simulink model "VSC_GFo_Fixed_Frequency_wi_LCL_v2017b"  (R2017b)
settings: Solver=ode1  StartTime=0.0  StopTime=10  FixedStep=Time_Step  MaxStep=1e-5  RelTol=1e-3
values from neighbouring files (symbols this model uses):
  fb = fn    (= 50)    [VSC_GFo_Init.m]    (also in VSC_GFo_Init_v1.m; VSC_GFo_Init_wi_LCL.m)
  fn = 50    [VSC_GFo_Init.m]    (also in VSC_GFo_Init_v1.m; VSC_GFo_Init_wi_LCL.m)
  GRD00_H = 5    [VSC_GFo_Init.m]    (also in VSC_GFo_Init_v1.m; VSC_GFo_Init_wi_LCL.m)
  GRD00_R = 4/100    (= 0.04)    [VSC_GFo_Init.m]    (also in VSC_GFo_Init_v1.m; VSC_GFo_Init_wi_LCL.m)
  GRD00_TD = 6    [VSC_GFo_Init.m]    (also in VSC_GFo_Init_v1.m = 2; VSC_GFo_Init_wi_LCL.m = 2)
  GRD00_TN = 1    [VSC_GFo_Init.m]    (also in VSC_GFo_Init_v1.m; VSC_GFo_Init_wi_LCL.m)
  GRD00_Ub = GRD00_Un    (= 400000)    [VSC_GFo_Init.m]    (also in VSC_GFo_Init_v1.m; VSC_GFo_Init_wi_LCL.m)
  Time_Step = 40e-6    (= 4e-05)    [VSC_GFo_Init.m]    (also in VSC_GFo_Init_v1.m; VSC_GFo_Init_wi_LCL.m)
  VSC01_Cf_pu = 0.066    [VSC_GFo_Init.m]    (also in VSC_GFo_Init_wi_LCL.m)
  VSC01_Lf_pu = 0.15    [VSC_GFo_Init.m]    (also in VSC_GFo_Init_wi_LCL.m)
  VSC01_Lt_pu = 0.15    [VSC_GFo_Init.m]    (also in VSC_GFo_Init_v1.m; VSC_GFo_Init_wi_LCL.m)
  VSC01_mp1 = 0.0043    [VSC_GFo_Init.m]    (also in VSC_GFo_Init_v1.m; VSC_GFo_Init_wi_LCL.m)
  VSC01_mp2 = 0.003    [VSC_GFo_Init.m]    (also in VSC_GFo_Init_v1.m = 0.0033; VSC_GFo_Init_wi_LCL.m = 0.0033)
  VSC01_mp3 = 0.04    [VSC_GFo_Init.m]    (also in VSC_GFo_Init_v1.m; VSC_GFo_Init_wi_LCL.m)
  VSC01_Pn = 1000 * 1e6    (= 1000000000)    [VSC_GFo_Init.m]    (also in VSC_GFo_Init_v1.m; VSC_GFo_Init_wi_LCL.m)
  VSC01_R = 4/100    (= 0.04)    [VSC_GFo_Init.m]    (also in VSC_GFo_Init_v1.m; VSC_GFo_Init_wi_LCL.m)
  VSC01_Rt_pu = 0.005    [VSC_GFo_Init.m]    (also in VSC_GFo_Init_v1.m; VSC_GFo_Init_wi_LCL.m)
  VSC01_Rv = 0.09    [VSC_GFo_Init.m]    (also in VSC_GFo_Init_v1.m; VSC_GFo_Init_wi_LCL.m)
  VSC01_Sn = VSC01_Pn/VSC01_cosPhi_n    [VSC_GFo_Init.m]    (also in VSC_GFo_Init_v1.m; VSC_GFo_Init_wi_LCL.m)
  VSC01_T1 = 0.121    [VSC_GFo_Init.m]    (also in VSC_GFo_Init_v1.m; VSC_GFo_Init_wi_LCL.m)
  VSC01_T2 = 0.022    [VSC_GFo_Init.m]    (also in VSC_GFo_Init_v1.m; VSC_GFo_Init_wi_LCL.m)
  VSC01_Tr_PLL = 0.010    (= 0.01)    [VSC_GFo_Init.m]    (also in VSC_GFo_Init_v1.m; VSC_GFo_Init_wi_LCL.m)
  VSC01_Udc_n = 640 * 1e3    (= 640000)    [VSC_GFo_Init.m]    (also in VSC_GFo_Init_v1.m; VSC_GFo_Init_wi_LCL.m)
  VSC01_Udcb = VSC01_Udc_n    (= 640000)    [VSC_GFo_Init.m]    (also in VSC_GFo_Init_v1.m; VSC_GFo_Init_wi_LCL.m)
  VSC01_Un1 = 320 * 1e3    (= 320000)    [VSC_GFo_Init.m]    (also in VSC_GFo_Init_v1.m; VSC_GFo_Init_wi_LCL.m)
  VSC01_Un2 = 400 * 1e3    (= 400000)    [VSC_GFo_Init.m]    (also in VSC_GFo_Init_v1.m; VSC_GFo_Init_wi_LCL.m)
  VSC01_W_LF = 60    [VSC_GFo_Init.m]    (also in VSC_GFo_Init_v1.m; VSC_GFo_Init_wi_LCL.m)
  VSC01_wc1 = wb/10    (= 31.4159265359)    [VSC_GFo_Init.m]    (also in VSC_GFo_Init_v1.m; VSC_GFo_Init_wi_LCL.m)
  VSC01_wc2 = 33.3    [VSC_GFo_Init.m]    (also in VSC_GFo_Init_v1.m; VSC_GFo_Init_wi_LCL.m)
  VSC01_wc3 = 2.5    [VSC_GFo_Init.m]    (also in VSC_GFo_Init_v1.m; VSC_GFo_Init_wi_LCL.m)
undefined symbols (not defined in the file or in its folder): C_line, VSC01_id0
libraries: powerlib x31, powerlib_meascontrol x1
(part 1 of 3)
settings Model: Creator=Frederic_Colas  LastModifiedBy=Frederic_Colas
settings OptimizationCC: LifeSpan=inf
settings DebuggingCC: UnconnectedInputMsg=none  UnconnectedOutputMsg=none  UnconnectedLineMsg=none  SFExecutionAtInitializationDiag=none
settings HardwareCC: ProdBitPerSizeT=32  ProdBitPerPtrDiffT=32  ProdWordSize=32  ProdHWDeviceType=Specified
settings CodeAppCC: StateflowObjectComments=on
settings SimscapeCC: SimscapeNormalizeSystem=off

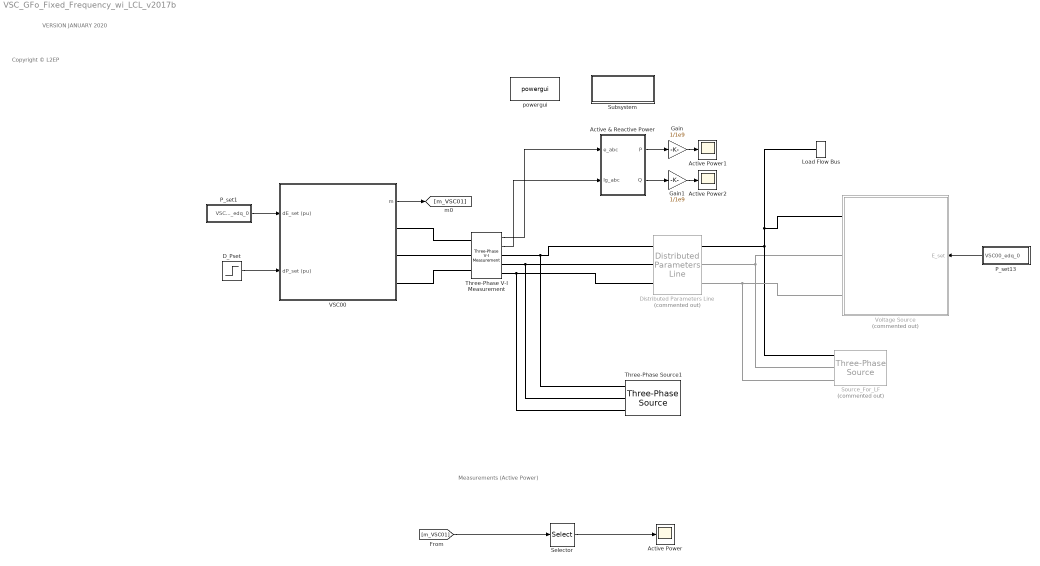
== system VSC_GFo_Fixed_Frequency_wi_LCL_v2017b ==
  note: VERSION JANUARY 2020
  note: Measurements (Active Power)
  note: Copyright © L2EP
  " Active & Reactive Power" : Subsystem  DialogController=POWERSYS.PowerSysDialog
  Active Power : Scope
  Active Power1 : Scope
  Active Power2 : Scope
  D_Pset : Step  Time=3  After=0.5  SampleTime=0
  Distributed Parameters Line : powerlib/Elements/Distributed Parameters Line  Commented=on  Phases=3  Frequency=50  Resistance=[0.01273 0.3864]  Inductance="[0.9337e-3  4.1264e-3]"  Capacitance=[12.74e-9 7.751e-9]  Length=50  x1=[-0.00032 2.39913762382152e-07 0 0;-0.00028 2.40449608965266e-07 0 0;-0.00024 2.40947485767745e-07 0 0;-0.0002 2.41407314169069e-07 189243.062485438 -353216.120618855;-0.00016 2.41829021557003e-07 193666.648507906 -350810.196287985;-0.00012 2.42212541339063e-07 198059.65232152 -348348.874960401;-8e-05 2.42557812953028e-07 202421.380220051 -345832.545307272;-4e-05 2.42864781876509e-07 206751.143436103 -343261.604686222]  x2=[-0.00032 -5.84182066675362e-12 0 0;-0.00028 -5.11361265966804e-12 0 0;-0.00024 -4.38459715386461e-12 0 0;-0.0002 -3.65488926934273e-12 177854.071673971 -358284.704095765;-0.00016 -2.92460423543639e-12 182342.2489454 -356021.494083621;-0.00012 -2.1938573726182e-12 186801.632261942 -353702.064150429;-8e-05 -1.46276407428886e-12 191231.517435277 -351326.780561063;-4e-05 -7.31439788555296e-13 195631.204935183 -348896.018400338]  x3=[-0.00032 -6.2867245833204e-11 0 0;-0.00028 -1.06466715946698e-10 0 0;-0.00024 -1.50049373731543e-10 0 0;-0.0002 -1.93608336980848e-10 284.201133471447 -561.76295681645;-0.00016 -2.37136727229364e-10 291.237829865103 -558.147319596773;-0.00012 -2.80627670839675e-10 298.228536429288 -554.443544445083;-8e-05 -3.24074300087621e-10 305.172149250395 -550.652216230411;-4e-05 -3.67469754246795e-10 312.067571851468 -546.773933647434]  x4=[-0.00032 3.8186796224243e-10 0 0;-0.00028 4.26357649227894e-10 0 0;-0.00024 4.70780009398051e-10 0 0;-0.0002 5.15128027947269e-10 998.290466477195 -2098.49155462395;-0.00016 5.59394701809321e-10 1024.58137422879 -2085.7813087356;-0.00012 6.03573040763248e-10 1050.71048870407 -2072.74169379946;-8e-05 6.47656068537197e-10 1076.67368381297 -2059.37476892188;-4e-05 6.91636823910058e-10 1102.46685966599 -2045.68264489526]  x5=0.000282770783497871  V1=ones(3,3)  V2=ones(3,3)  I1=ones(3,3)  I2=ones(3,3)  nHarmo=1  Measurements=None
      settings: SourceProductName=Simscape Power Systems
  Gain : Gain  Gain=1/1e9
  Gain1 : Gain  Gain=1/1e9
  Load Flow Bus : powerlib/Measurements/Load Flow Bus  LConnTagsString=a  Phases=single  Connectors=on one side  ID=BUS_1  Vbase=400000  Vref=1  Vangle=0  VLF=1  VLFb=1  VLFc=1  angleLF=0  angleLFb=0  angleLFc=0
      settings: SourceProductName=Simscape Electrical
  P_set1 : Subsystem
  P_set13 : Subsystem
  Selector : Selector  InputPortWidth=3  IndexOptions=Index vector (dialog)  Indices=[1]  OutputSizes=1
  Source_For_LF : powerlib/Electrical Sources/Three-Phase Source  Commented=on  InternalConnection=Yg  VoltagePhases=off  Voltage=(400000)*1  PhaseAngle=0  Voltage_phases=[25e3 25e3 25e3]/sqrt(3)  PhaseAngles_phases=[0 -120 +120]  Frequency=fb  NonIdealSource=on  SpecifyImpedance=off  Resistance=0  Inductance=0  ShortCircuitLevel=100e6  BaseVoltage=GRD00_Un  XRratio=7  BusType=swing  Pref=P0  Qref=Q0  Prefabc=[10e3, 10e3, 10e3]  Qrefabc=[0, 0, 0]  Qmin=-inf  Qmax=inf
      settings: SourceProductName=Simscape Electrical
  Subsystem : Subsystem
      settings: OpenFcn=LoadFlow_VSC
      mask Display: color('blue'),disp('Update Loadflow')
  Three-Phase V-I Measurement : powerlib/Measurements/Three-Phase V-I Measurement  VoltageMeasurement=phase-to-ground  SetLabelV=off  LabelV=Vabc  Vpu=off  VpuLL=off  CurrentMeasurement=yes  SetLabelI=off  LabelI=Iabc  Ipu=off  Pbase=100e6  Vbase=500e3  OutputType=Complex  PhasorSimulation=off  PSBequivalent=0
  Three-Phase Source1 : powerlib/Electrical Sources/Three-Phase Source  InternalConnection=Yg  VoltagePhases=off  Voltage=(400000)*1  PhaseAngle=0  Voltage_phases=[25e3 25e3 25e3]/sqrt(3)  PhaseAngles_phases=[0 -120 +120]  Frequency=50  NonIdealSource=off  SpecifyImpedance=off  Resistance=0.8929  Inductance=16.58e-3  ShortCircuitLevel=100e6  BaseVoltage=25e3  XRratio=7  BusType=swing  Pref=10e3  Qref=0  Prefabc=[10e3, 10e3, 10e3]  Qrefabc=[0, 0, 0]  Qmin=-inf  Qmax=inf
  VSC00 : Subsystem  mask(VSC){fb=fb, Sn=VSC01_Sn, Pn=VSC01_Pn, Un1=VSC01_Un1, Un2=VSC01_Un2, Rt_pu=VSC01_Rt_pu, Lt_pu=VSC01_Lt_pu, Lm_pu=500, Rm_pu=500, Lf_pu=0.15, Cf_pu=0.066, Tr_PLL=VSC01_Tr_PLL, Tr_i=0, D_i=0, Tr_v=0, D_v=0, Val_Freq_Support=on, R_percent=VSC01_R, Rv=VSC01_Rv, W_TVR=VSC01_W_LF, gainpopup=2, wc1=VSC01_wc1, mp1=VSC01_mp1, wc2=VSC01_wc2, mp2=VSC01_mp2, wc3=VSC01_wc3, mp3=VSC01_mp3, T1=VSC01_T1, T2=VSC01_T2, LFpopup=PQ, P0=0.3, Q0=0, V0=1, Theta0=0}
      mask prompts: fb "Nominal Frequency (Hz)"; Sn "Nominal Apparent Power (VA)"; Pn "Nominal Power (W)"; Un1 "VSC side Nominal Ph-Ph Voltage (V)"; Un2 "Grid side Nominal Ph-Ph Voltage (V)"; Rt_pu "R (pu)"; Lt_pu "L (pu)"; Lm_pu "Rm (pu)"; Rm_pu "Lm (pu)"; Lf_pu "Lf (pu)"; Cf_pu "Cf (pu)"; Tr_PLL "PLL Time response (s)"; Tr_i "Time Response (s)"; D_i "Damping factor"; Tr_v "Time Response (s)"; D_v "Damping factor"; Val_Freq_Support "Frequency Support"; R_percent "Droop Gain (%)"; Rv "Damping Resistance (Rv)"; W_TVR "Dr filter"; gainpopup "Strategy"; wc1 "wc"; mp1 "mp"; wc2 "wc"; mp2 "mp"; wc3 "wc"; mp3 "mp"; P0 "Initial Active Power (pu)"; Q0 "Initial Reactive Power (pu)"; V0 "Initial Voltage (pu)"; Theta0 "Initial Angle (°)"
      mask init:
      | % Update Name of LF bus for internal purpose
      |     NameStr = [get_param(gcb,'Name')];% '_LF'];
      |     set_param([gcb '/Load Flow Bus'],'ID',NameStr);
      |     %disp(NameStr);
      |     
      | % Increase size of Mask dialog box
      |    % pause(0.1);
      |     
      |     
      | % Base values
      |     %Un = Un1;
      |     Pb = Pn;
      |     cos_phi_n = Pn/Sn;
      |     Sb = Pb/cos_phi_n;
      |     %Ub = Un;
      |     Vn = Un1/sqrt(3);
      |     Vb = Vn;
      |     Vn2 = Un2/sqrt(3);
      |     Vb2=Vn2;
      |     %Ib = Sb / Ub;
      |     Ib = Sb / (3*Vb);
      |     wb = 2*pi*fb;
      |     Zb = (Vb*sqrt(3))^2 / Sb;
      |     Lb = Zb / wb; % Inductance base value
      |     Cb = 1 / (Zb*wb); 
      |   
      | % PLL derivation of the parameters
      |     wn_PLL=5/Tr_PLL;
      |     zeta_PLL = 1;
      |     Kp_PLL_pu = 2*zeta_PLL*wn_PLL/wb;
      |     Ki_PLL_pu = wn_PLL^2/wb;
      | 
      |  %% Inner controller: Current & Voltage 
      | % Current PI controller   
      |     Tr_i = 5 * 1e-3;                    % Time response [s]
      |     D_i = 0.707;                        % Damping factor
      |     Kp_i = 0.73001;                     % Proportional current gain
      |     Ki_i = 1.19073;                     % Integral current gain
      |     Ti_i = Kp_i / Ki_i;
      |     
      |     Kffi = 1;                           % Current feed forward (enabled)  
      |  % Voltage PI controller   
      |     Tr_v = 5 * 1e-3;                    % Time response [s]
      |     D_v = 0.707;                        % Damping factor
      |     Kp_v = 0.52001;                     % Proportional current gain
      |     Ki_v = 1.16073;                     % Integral current gain
      |     Ti_iv = Kp_v / Ki_v;  
      |     Kffv = 1;                           % Current feed forward (enabled)     
      | % Set the chosen strategy
      |     Chosen_Strategy = str2double(gainpopup);
      |     
      | % Set the frequency droop gain
      |     R = R_percent;
      | 
      | % Compute Initial Voltage of VSC 
      | %   from steady-state output transformer model and Loadflow result
      |     if (LFpopup == 'PQ')
      |         V0 = 1;
      |     end
      | %%%%%%%%%%%%%%%%%%%        
      | %     R1_pu = Rt_pu/2;
      | %     L1_pu = Lt_pu/2;
      | %     R2_pu = Rt_pu/2;
      | %     L2_pu = Lt_pu/2;
      | %     X1_pu = L1_pu;
      | %     X2_pu = L2_pu;
      | %     Xm_pu = Lm_pu;
      | %     Zm_pu = 1/(1/Rm_pu+1/(1i*Xm_pu));
      | %     S0=P0+1i*Q0;
      | %     I2 = conj(S0)/(V0);
      | %     Vm = (R2_pu+1i*X2_pu)*I2 + V0;
      | %     Im = Vm/Zm_pu;
      | %     I1 = I2 + Im;
      | %     V1 = (R1_pu+1i*X1_pu) * I1 + Vm;
      | %     Vvsc0 = abs(V1);
      | %    % disp(Vvsc0*1000)
      | %     Theta_vsc0 = angle(V1) * 180/pi+Theta0;
      | %%%%%%%%%%%%%%%%%%%
      | %Rf_pu=0.005;
      | %Lf_pu=0.15;
      | %Cf_pu = 0.066;
      | %%%%%%%%%%%%%%%%%%%        
      |     R1_pu = (Rt_pu/2) ;
      |     L1_pu = (Lt_pu/2);
      |     R2_pu = Rt_pu/2;
      |     L2_pu = Lt_pu/2;
      |     X1_pu = L1_pu;
      |     X2_pu = L2_pu;
      |     Xm_pu = Lm_pu;
      |     Xc_pu = Cf_pu;
      |     Xf_pu = Lf_pu;
      |     Zt_pu = 1/(1/Rm_pu+1/(1i*Xm_pu));
      |     Zc_pu = 1/(1i*Xc_pu);
      |     S0=P0+1i*Q0; % Apparent output Power
      |     I2 = conj(S0)/(V0); % Output current
      |     %Vm = (R2_pu+1i*X2_pu)*I2 + V0;
      |     Vt = (R2_pu+1i*X2_pu) * I2 + V0; % Magnetizing Voltage
      |     %Vcf = (R2_pu+1i*X2_pu)*I2 + V0;
      |     It = Vt/Zt_pu; % Magnetizing current
      |     I1 = I2 + It; % output transformer Primary side current
      |     V1 = (R1_pu+1i*X1_pu) * I1 + Vt; % Output transformer Primary voltage = output capacitor voltage
      |     abs(V1)
      |     
      |     %LC Filter
      |     Im = I1 + 1i*Xc_pu*V1; % Converter output current
      |     Imd0 = abs(Im)*cos(angle(Im)-angle(V1));
      |     Imq0 = abs(Im)*sin(angle(Im)-angle(V1));
      |     Vm = 1i*Xf_pu*Im + V1; % Converter initial output voltage
      |     %Icf = Vcf/Zc_pu;
      |     %I1 = -It + Icf;
      |     %V1 = (Rf_pu+1i*Xf_pu) * I1 + Vcf;
      |     Vmd0 = abs(Vm)*cos(angle(Vm)-angle(V1));
      |     Vmq0 = abs(Vm)*sin(angle(Vm)-angle(V1));
      |     
      |     %Filtre LC
      |     
      |     Vvsc0 = abs(Vm)
      |     Theta_vsc0 = angle(Vm) * 180/pi+Theta0;
      | %%%%%%%%%%%%%%%%%%%
      | 
      | 
      |     %vd0=Vvsc0*cos(Theta0*2*pi/180);
      |     %vq0=Vvsc0*sin(Theta0*2*pi/180); 
      |  
      |     %Va0 = Vvsc0*sqrt(2)*Ub/sqrt(3)*sin(Theta_vsc0*pi/180);
      |     %Vb0 = Vvsc0*sqrt(2)*Ub/sqrt(3)*sin(Theta_vsc0*pi/180-2*pi/3);
      |     %Vc0 = Vvsc0*sqrt(2)*Ub/sqrt(3)*sin(Theta_vsc0*pi/180+2*pi/3);
      |     
      |     Va0 = Vvsc0*sqrt(2)*Vb*sin(Theta_vsc0*pi/180);
      |     Vb0 = Vvsc0*sqrt(2)*Vb*sin(Theta_vsc0*pi/180-2*pi/3);
      |     Vc0 = Vvsc0*sqrt(2)*Vb*sin(Theta_vsc0*pi/180+2*pi/3);
      |     
      | % Generate string to display LF results on Mask
      |     %str_tmp = fprintf("Vvsc0 = %d, Theta_vsc0 = %d°",Vvsc0,Theta_vsc0);
      |     mo = get_param(gcb,'MaskObject');
      |     mo.getDialogControl('LF_vsc_str').Prompt = ['V0 = ', num2str(Vvsc0),' pu, Angle = ', num2str(Theta_vsc0),'°'];
      |     mo.getDialogControl('LF_pcc_str').Prompt = ['V0 = ', num2str(V0),' pu, Angle = ', num2str(Theta0),'°'];
      |     mo.getDialogControl('LF_pcc_Power_str').Prompt = ['P0 = ', num2str(P0),' pu, Q0 = ', num2str(Q0),' pu'];
      |     %set_param([gcb],'LF_str',str_tmp);
      |  %GRD00_Theta0 = Theta0;
      |  %P0 = 200e6;
      |  %Q0 = 0;
      |  % Initial current values of VSC (dq pu) 
      |  %id0 =(P0*vd0+Q0*vq0)/(vd0^2+vq0^2) * 1/Ib; %
      |  %iq0 =(P0*vq0-Q0*vd0)/(vd0^2+vq0^2) * 1/Ib; %Initial current in the connexion inductance
      settings: OpenFcn=|
      | NameStr = get_param(gcb,'Name');
      | open_system(gcbh, 'Mask');
      | 
      | h2AllOpenDlgs = DAStudio.ToolRoot.getOpenDialogs;
      | 
      | for i=1:length(h2AllOpenDlgs)
      |     try
      |          %disp(h2AllOpenDlgs(i).getSource.getBlock.Name);
      |         Dialog_block_name = h2AllOpenDlgs(i).getSource.getBlock.Name;
      |          %strcmp(Dialog_block_name, NameStr),
      |         if (strcmp(h2AllOpenDlgs(i).getSource.getBlock.Name, NameStr))
      |             iPos = h2AllOpenDlgs(i).position;
      |             h2AllOpenDlgs(i).position = [iPos(1)   iPos(2)   iPos(3)*1.5   iPos(4)];
      |         end
      |     end
      | end
      mask TypeOptions gainpopup: 1 | 2 | 3
      mask Callback gainpopup:
      | % Get the mask parameter values. This is a cell
      | %   array of character vectors.
      | maskStr = get_param(gcb,'gainpopup');
      | p=Simulink.Mask.get(gcb);
      | 
      | % The pop-up menu is the first mask parameter.
      | %   Check the value selected in the pop-up
      | if strcmp(maskStr,'1'),
      | 
      |     % Set the visibility of both parameters on when
      |     %   User-defined is selected in the pop-up.
      |     p.getDialogControl('Param_Strat_1').Visible='on';
      |     p.getDialogControl('Param_Strat_2').Visible='off';
      |     p.getDialogControl('Param_Strat_3').Visible='off';
      | 
      | elseif strcmp(maskStr,'2'),
      | 
      |     % Set the visibility of both parameters on when
      |     %   User-defined is selected in the pop-up.
      |     p.getDialogControl('Param_Strat_1').Visible='off';
      |     p.getDialogControl('Param_Strat_2').Visible='on';
      |     p.getDialogControl('Param_Strat_3').Visible='off';
      | 
      |     % Turn off the visibility of the Value field
      |     %   when User-defined is not selected.
      | else
      | 
      |     % Set the visibility of both parameters on when
      |     %   User-defined is selected in the pop-up.
      |     p.getDialogControl('Param_Strat_1').Visible='off';
      |     p.getDialogControl('Param_Strat_2').Visible='off';
      |     p.getDialogControl('Param_Strat_3').Visible='on';
      | 
      | end
      mask TypeOptions LFpopup: Swing | PQ | PV
      mask Callback LFpopup:
      | % Get the mask parameter values. This is a cell
      | %   array of character vectors.
      | maskStr = get_param(gcb,'LFpopup');
      | p=Simulink.Mask.get(gcb);
      | 
      | % The pop-up menu is the first mask parameter.
      | %   Check the value selected in the pop-up
      | if strcmp(maskStr,'Swing'),
      | 
      |     % Set the visibility of both parameters on when
      |     %   User-defined is selected in the pop-up.
      |     p.getParameter('P0').Visible='off';
      |     p.getParameter('Q0').Visible='off';
      |     p.getParameter('V0').Visible='on';
      |     p.getParameter('Theta0').Visible='on';
      |     set_param([gcb '/Source_For_LF'],'BusType','swing');
      | 
      | elseif strcmp(maskStr,'PQ'),
      | 
      |     % Set the visibility of both parameters on when
      |     %   User-defined is selected in the pop-up.
      |     p.getParameter('P0').Visible='on';
      |     p.getParameter('Q0').Visible='on';
      |     p.getParameter('V0').Value='1';
      |     set_param(gcb,'V0','1');
      |     p.getParameter('V0').Visible='off';
      |     p.getParameter('Theta0').Visible='off';
      |     set_param([gcb '/Source_For_LF'],'BusType','PQ');
      | 
      |     % Turn off the visibility of the Value field
      |     %   when User-defined is not selected.
      | else
      | 
      |     % Set the visibility of both parameters on when
      |     %   User-defined is selected in the pop-up.
      |     p.getParameter('P0').Visible='on';
      |     p.getParameter('Q0').Visible='off';
      |     p.getParameter('V0').Visible='on';
      |     p.getParameter('Theta0').Visible='off';
      |     set_param([gcb '/Source_For_LF'],'BusType','PV');
      | 
      | end
      mask DialogControl Nominal_Param Prompt: Nominal Value
      mask DialogControl Container20 Prompt: Output Transformer
      mask DialogControl Container26 Prompt: Output Filter
      mask DialogControl Control_Param Prompt: Control Parameter
      mask DialogControl Container13 Prompt: Inner Control Parameters
      mask DialogControl Container27 Prompt: Current Loop
      mask DialogControl Container29 Prompt: Voltage Loop
      mask DialogControl Container14 Prompt: Frequency Support
      mask DialogControl Container15 Prompt: Transient Virtual Resistor
      mask DialogControl Container18 Prompt: Control Strategy
      mask DialogControl Title_Strat_1 Prompt: Strategy 1
      mask DialogControl Title_Strat_2 Prompt: Strategy 2
      mask DialogControl Title_Strat_3 Prompt: Strategy 3
      mask DialogControl LF_Param Prompt: Loadflow
      mask DialogControl Control4 Prompt: Initial Operating Point
      mask DialogControl Container24 Prompt: VSC side
      mask DialogControl LF_vsc_str Prompt: V0 = 0.9961 pu, Angle = 5.1844°
      mask DialogControl Container25 Prompt: PCC
      mask DialogControl LF_pcc_str Prompt: V0 = 1 pu, Angle = 0°
      mask DialogControl LF_pcc_Power_str Prompt: P0 = 0.3 pu, Q0 = 0 pu
      mask DialogControl UpdateLoadflow Prompt: Update Loadflow
      mask DialogControl UpdateLoadflow Callback: Load_Flow_VSC
  Voltage Source : Subsystem  Commented=on  mask(Inertial_Voltage_source){fb=fb, Sc=1e9, Ub=GRD00_Ub, H_eq=GRD00_H, Droop=GRD00_R, TN=GRD00_TN, TD=GRD00_TD}
      mask prompts: fb "Nominal Frequency (Hz)"; Sc "Nominal Power (VA)"; Ub "Nominal Voltage (V)"; H_eq "Inertial Constant H (s)"; Droop "Droop Gain"; TN "Lead Time Constant"; TD "Lag Time Constant"
      mask init:
      | % Base values
      |     wb=2*pi*fb;
      |     Ib=Sc/(sqrt(3)*Ub);
      |     Vb=Ub/sqrt(3);
      |     e0=Vb;
      |     Theta_e0=0;
      |   
      | % Parameters
      |     R=Droop;
      mask DialogControl Container5 Prompt: Nominal Values
      mask DialogControl Container16 Prompt: Network Time Constants
  powergui : powerlib/powergui  Priority=1  SimulationMode=Discrete  SampleTime=Time_Step  frequency=60  Iterations=100  frequencyindice=50  Pbase=1000e6  ErrMax=1e-5  UnitsV=kV  UnitsW=MW  buscounter=0  FunctionMessages=off  echomessages=off  EnableUseOfTLC=off  CurrentSourceSwitches=off  DisableSnubberDevices=off  DisableRonSwitches=off  DisableVfSwitches=off  DisplayEquations=off  SolverType=Tustin/Backward Euler (TBE)  Interpol=off  ExternalGateDelay=off  methode=off  Ts=100  x0status=blocks  SPID=on  SwTol=0  HookPort=off  RestoreLinks=warning  ResistiveCurrentMeasurement=off  Frange=[0:2:500]  Ylog=off  Xlog=on  ShowGrid=off  save=off  variable=ZData  structure=0  ZoomFFT=off  StartTime=0.0  cycles=1  DisplayStyle=1  fundamental=60  FreqAxis=off  MaxFrequency=1000  frequencyindicesteady=1  RmsSteady=1  display=off
  wires:
  P_set1/1(VSC01_edq_0) -> VSC00/1(dE_set (pu))
  D_Pset/1 -> VSC00/2(dP_set (pu))
  [m_VSC01] -> Selector/1
  P_set13/1(VSC00_edq_0) -> Voltage Source/1(E_set)
  Selector/1 -> Active Power/1
  VSC00/1(m) -> [m_VSC01]
  Three-Phase V-I Measurement/1 -> " Active & Reactive Power"/1(e_abc)
  Three-Phase V-I Measurement/2 -> " Active & Reactive Power"/2(Ig_abc)
  " Active & Reactive Power"/1(P) -> Gain/1
  " Active & Reactive Power"/2(Q) -> Gain1/1
  Gain/1 -> Active Power1/1
  Gain1/1 -> Active Power2/1
  connections:
  Source_For_LF/RConn2 -- Voltage Source/RConn2 -- Distributed Parameters Line/RConn2
  Voltage Source/RConn1 -- Source_For_LF/RConn1 -- Distributed Parameters Line/RConn1 -- Load Flow Bus/LConn1
  Source_For_LF/RConn3 -- Distributed Parameters Line/RConn3 -- Voltage Source/RConn3
  Three-Phase V-I Measurement/LConn2 -- VSC00/RConn2
  Three-Phase V-I Measurement/RConn2 -- Three-Phase Source1/RConn2 -- Distributed Parameters Line/LConn2
  Three-Phase V-I Measurement/RConn1 -- Distributed Parameters Line/LConn1 -- Three-Phase Source1/RConn1
  Three-Phase V-I Measurement/RConn3 -- Distributed Parameters Line/LConn3 -- Three-Phase Source1/RConn3
  Three-Phase V-I Measurement/LConn3 -- VSC00/RConn3
  Three-Phase V-I Measurement/LConn1 -- VSC00/RConn1

== system VSC_GFo_Fixed_Frequency_wi_LCL_v2017b/ Active & Reactive Power ==
  e_abc : Inport  PortDimensions=3
  Ig_abc : Inport  Port=2  PortDimensions=3
  Demux : Demux  Outputs=3
  Mux : Mux  Inputs=3
  Product1 : Product  SaturateOnIntegerOverflow=on  InputSameDT=on  OutDataTypeStr=Inherit: Same as first input
  Product3 : Product  SaturateOnIntegerOverflow=on  InputSameDT=on  OutDataTypeStr=Inherit: Same as first input
  Sum : Sum  Inputs=+-  SaturateOnIntegerOverflow=on  InputSameDT=on  OutDataTypeStr=Inherit: Same as first input
  Sum1 : Sum  Inputs=1  SaturateOnIntegerOverflow=on  InputSameDT=on  OutDataTypeStr=Inherit: Same as first input
  Sum4 : Sum  Inputs=1  SaturateOnIntegerOverflow=on  InputSameDT=on  OutDataTypeStr=Inherit: Same as first input
  Sum5 : Sum  Inputs=+-  SaturateOnIntegerOverflow=on  InputSameDT=on  OutDataTypeStr=Inherit: Same as first input
  Sum6 : Sum  Inputs=+-  SaturateOnIntegerOverflow=on  InputSameDT=on  OutDataTypeStr=Inherit: Same as first input
  pu->V : Gain  Gain=1/sqrt(3)  SaturateOnIntegerOverflow=on  OutDataTypeStr=Inherit: Same as input  ParamDataTypeStr=Inherit: Same as input
  P : Outport
  Q : Outport  Port=2
  wires:
  pu->V/1 -> Q/1  "Q"
  Mux/1 -> Product3/1
  Sum6/1 -> Mux/2
  Sum5/1 -> Mux/1
  Sum/1 -> Mux/3
  Demux/3 -> Sum6/1, Sum5/2
  Demux/2 -> Sum5/1, Sum/2
  Demux/1 -> Sum6/2, Sum/1
  Sum4/1 -> P/1  "P"
  Ig_abc/1 -> Product3/2, Product1/2
  e_abc/1 -> Demux/1, Product1/1
  Product1/1 -> Sum4/1
  Product3/1 -> Sum1/1
  Sum1/1 -> pu->V/1

== system VSC_GFo_Fixed_Frequency_wi_LCL_v2017b/P_set1 ==
  Mux : Mux  Inputs=2
  ed0 : Constant  Value=0
  eq0 : Constant  Value=0
  VSC01_edq_0 : Outport
  wires:
  eq0/1 -> Mux/2
  ed0/1 -> Mux/1
  Mux/1 -> VSC01_edq_0/1

== system VSC_GFo_Fixed_Frequency_wi_LCL_v2017b/P_set13 ==
  Mux : Mux  Inputs=2
  ed1 : Constant  Value=0
  eq1 : Constant
  VSC00_edq_0 : Outport
  wires:
  Mux/1 -> VSC00_edq_0/1
  eq1/1 -> Mux/1
  ed1/1 -> Mux/2

== system VSC_GFo_Fixed_Frequency_wi_LCL_v2017b/Subsystem ==

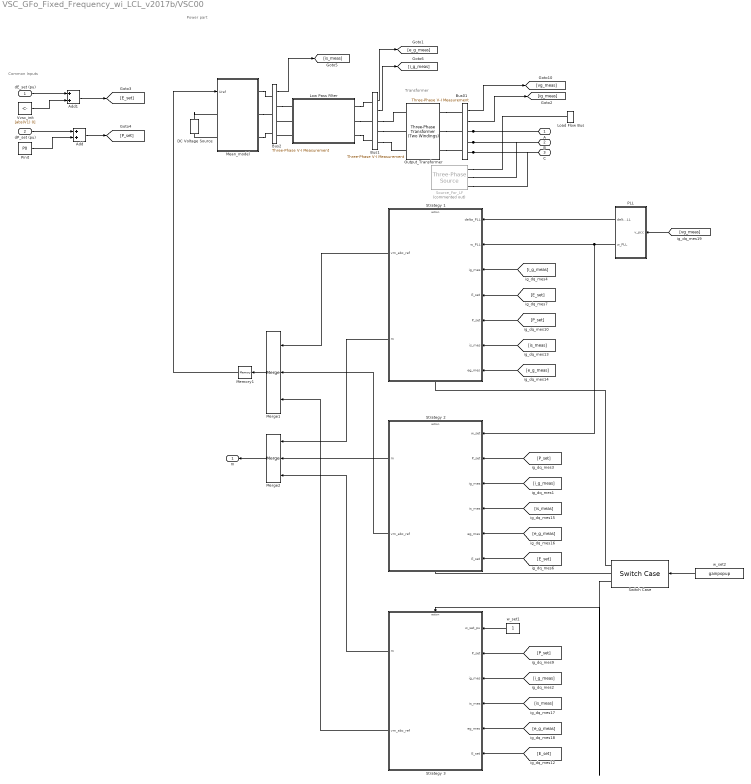
== system VSC_GFo_Fixed_Frequency_wi_LCL_v2017b/VSC00 ==
  note: Power part
  note: Common Inputs
  note: Transformer
  dE_set (pu) : Inport
  dP_set (pu) : Inport  Port=2
  Add : Sum
  Add1 : Sum
  Bus01 : powerlib/Measurements/Three-Phase V-I Measurement  VoltageMeasurement=phase-to-ground  SetLabelV=off  LabelV=Vabc  Vpu=off  VpuLL=off  CurrentMeasurement=yes  SetLabelI=off  LabelI=Iabc  Ipu=off  Pbase=100e6  Vbase=500e3  OutputType=Complex  PhasorSimulation=off  PSBequivalent=0
      settings: SourceProductName=Simscape Electrical
  Bus1 : powerlib/Measurements/Three-Phase V-I Measurement  VoltageMeasurement=phase-to-ground  SetLabelV=off  LabelV=Vabc  Vpu=off  VpuLL=off  CurrentMeasurement=yes  SetLabelI=off  LabelI=Iabc  Ipu=off  Pbase=100e6  Vbase=500e3  OutputType=Complex  PhasorSimulation=off  PSBequivalent=0
      settings: SourceProductName=Simscape Electrical
  Bus2 : powerlib/Measurements/Three-Phase V-I Measurement  VoltageMeasurement=no  SetLabelV=off  LabelV=Vabc  Vpu=off  VpuLL=off  CurrentMeasurement=yes  SetLabelI=off  LabelI=Iabc  Ipu=off  Pbase=100e6  Vbase=500e3  OutputType=Complex  PhasorSimulation=off  PSBequivalent=0
      settings: SourceProductName=Simscape Electrical
  DC Voltage Source : powerlib/Electrical Sources/DC Voltage Source  Amplitude=VSC01_Udc_n  Measurements=Voltage
      settings: SourceProductName=Simscape Electrical
  Load Flow Bus : powerlib/Measurements/Load Flow Bus  LConnTagsString=a  Phases=single  Connectors=on one side  ID=VSC00  Vbase=Un2  Vref=V0  Vangle=Theta0  VLF=1.002  VLFb=1  VLFc=1  angleLF=1.777  angleLFb=0  angleLFc=0
      settings: SourceProductName=Simscape Electrical
  Low Pass Filter : Subsystem
  Mean_model : Subsystem
  Memory1 : Memory  InitialCondition=[Va0 Vb0 Vc0]
  Merge1 : Merge  Inputs=3
  Merge2 : Merge  Inputs=3
  Output_Transformer : powerlib/Elements/Three-Phase Transformer (Two Windings)  Winding1Connection=Yg  Winding2Connection=Yg  CoreType=Three single-phase transformers  SetSaturation=off  Hysteresis=off  DataFile='hysteresis'  SetInitialFlux=off  Measurements=None  UNITS=pu  NominalPower=[Sn , fn ]  Winding1=[Un1 , Rt_pu/2 , Lt_pu/2]  Winding2=[Un2 , Rt_pu/2 , Lt_pu/2]  Rm=Rm_pu  Lm=Lm_pu  L0=0.5  Saturation=[ 0,0 ; 0.0024,1.2 ; 1.0,1.52 ]  InitialFluxes=[ 0.8 , -0.8 , 0.7 ]  MoreParameters=off  BreakLoop=off  DataType=off  TransfoNumber=1
      settings: SourceProductName=Simscape Electrical
  PLL : Subsystem
  Pinit : Constant  Value=P0
  Source_For_LF : powerlib/Electrical Sources/Three-Phase Source  Commented=on  InternalConnection=Yg  VoltagePhases=off  Voltage=(400000)*1.00234  PhaseAngle=1.7773  Voltage_phases=[25e3 25e3 25e3]/sqrt(3)  PhaseAngles_phases=[0 -120 +120]  Frequency=50  NonIdealSource=off  SpecifyImpedance=off  Resistance=0  Inductance=0  ShortCircuitLevel=100e6  BaseVoltage=Un  XRratio=7  BusType=PQ  Pref=P0*Sb  Qref=Q0*Sb  Prefabc=[10e3, 10e3, 10e3]  Qrefabc=[0, 0, 0]  Qmin=-inf  Qmax=inf
      settings: SourceProductName=Simscape Electrical
  Strategy 1 : Subsystem
  Strategy 2 : Subsystem
  Strategy 3 : Subsystem
  Switch Case : SwitchCase  CaseConditions={1,2,3}  ShowDefaultCase=off
  Vvsc_init : Constant  Value=[abs(V1) 0]
  w_set1 : Constant
  w_set2 : Constant  Value=gainpopup
  A : PMIOPort  Port=1  Side=Right
  B : PMIOPort  Port=2  Side=Right
  C : PMIOPort  Port=3  Side=Right
  m : Outport
  wires:
  PLL/1(delta_PLL) -> Strategy 1/1(delta_PLL)
  w_set1/1 -> Strategy 3/1(w_set_pu)
  Add/1 -> [P_set]
  Strategy 2/1(m) -> Merge2/2
  [i_g_meas] -> Strategy 1/3(ig_mes)
  Switch Case/1 -> Strategy 1/Action
  [vg_meas] -> PLL/1(v_pcc)
  Merge2/1 -> m/1
  Bus01/2 -> [ig_meas]
  dE_set (pu)/1 -> Add1/1
  Strategy 1/1(vm_abc_ref) -> Merge1/1
  Switch Case/3 -> Strategy 3/Action
  Strategy 1/2(m) -> Merge2/1
  w_set2/1 -> Switch Case/1
  Bus01/1 -> [vg_meas]
  [P_set] -> Strategy 3/2(P_set)
  Strategy 3/1(m) -> Merge2/3
  PLL/2(w_PLL) -> Strategy 2/1(w_set), Strategy 1/2(w_PLL)
  Add1/1 -> [E_set]
  [P_set] -> Strategy 2/2(P_set)
  Strategy 2/2(vm_abc_ref) -> Merge1/2
  Vvsc_init/1 -> Add1/2
  Merge1/1 -> Memory1/1
  [P_set] -> Strategy 1/5(P_set)
  Pinit/1 -> Add/2
  Switch Case/2 -> Strategy 2/Action
  dP_set (pu)/1 -> Add/1
  [E_set] -> Strategy 1/4(E_set)
  Memory1/1 -> Mean_model/1(Uref)
  Bus1/1 -> [e_g_meas]
  Bus2/1 -> [is_meas]
  [e_g_meas] -> Strategy 1/7(eg_mes)
  [is_meas] -> Strategy 1/6(is_mes)
  Bus1/2 -> [i_g_meas]
  [E_set] -> Strategy 2/6(E_set)
  [e_g_meas] -> Strategy 2/5(eg_mes)
  [is_meas] -> Strategy 2/4(is_mes)
  [i_g_meas] -> Strategy 2/3(ig_mes)
  [i_g_meas] -> Strategy 3/3(ig_mes)
  [is_meas] -> Strategy 3/4(is_mes)
  [e_g_meas] -> Strategy 3/5(eg_mes)
  [E_set] -> Strategy 3/6(E_set)
  Strategy 3/2(vm_abc_ref) -> Merge1/3
  connections:
  Bus01/RConn3 -- C/RConn1 -- Source_For_LF/RConn3
  Bus01/RConn1 -- Load Flow Bus/LConn1 -- A/RConn1 -- Source_For_LF/RConn1
  Bus01/RConn2 -- B/RConn1 -- Source_For_LF/RConn2
  Output_Transformer/RConn3 -- Bus01/LConn3
  DC Voltage Source/RConn1 -- Mean_model/LConn1
  Output_Transformer/RConn2 -- Bus01/LConn2
  Output_Transformer/RConn1 -- Bus01/LConn1
  Bus1/RConn3 -- Output_Transformer/LConn3
  Bus1/RConn2 -- Output_Transformer/LConn2
  Bus1/RConn1 -- Output_Transformer/LConn1
  Mean_model/RConn3 -- Bus2/LConn3
  Mean_model/RConn2 -- Bus2/LConn2
  Mean_model/RConn1 -- Bus2/LConn1
  Low Pass Filter/RConn1 -- Bus1/LConn1
  Low Pass Filter/RConn2 -- Bus1/LConn2
  Low Pass Filter/RConn3 -- Bus1/LConn3
  Bus2/RConn1 -- Low Pass Filter/LConn1
  Low Pass Filter/LConn2 -- Bus2/RConn2
  Low Pass Filter/LConn3 -- Bus2/RConn3
  Mean_model/LConn2 -- DC Voltage Source/LConn1

== system VSC_GFo_Fixed_Frequency_wi_LCL_v2017b/Voltage Source ==
  E_set : Inport
  Load Flow Bus : powerlib/Measurements/Load Flow Bus  LConnTagsString=a  Phases=single  Connectors=on one side  ID=BUS_1  Vbase=Ub  Vref=1  Vangle=0  VLF=1  VLFb=1  VLFc=1  angleLF=0  angleLFb=0  angleLFc=0
      settings: SourceProductName=Simscape Electrical
  Mean_model : Subsystem  Commented=on
  Source_For_LF : powerlib/Electrical Sources/Three-Phase Source  InternalConnection=Yg  VoltagePhases=off  Voltage=(400000)*1  PhaseAngle=0  Voltage_phases=[25e3 25e3 25e3]/sqrt(3)  PhaseAngles_phases=[0 -120 +120]  Frequency=fb  NonIdealSource=on  SpecifyImpedance=off  Resistance=0  Inductance=0  ShortCircuitLevel=100e6  BaseVoltage=GRD00_Un  XRratio=7  BusType=swing  Pref=P0  Qref=Q0  Prefabc=[10e3, 10e3, 10e3]  Qrefabc=[0, 0, 0]  Qmin=-inf  Qmax=inf
      settings: SourceProductName=Simscape Electrical
  Voltage generation : Subsystem
  A : PMIOPort  Port=1  Side=Right
  B : PMIOPort  Port=2  Side=Right
  C : PMIOPort  Port=3  Side=Right
  wires:
  E_set/1 -> Voltage generation/1(E_set)
  Voltage generation/1(vg_abc) -> Mean_model/1(u_abc)
  connections:
  Mean_model/RConn3 -- C/RConn1 -- Source_For_LF/RConn3
  Mean_model/RConn2 -- B/RConn1 -- Source_For_LF/RConn2
  Mean_model/RConn1 -- A/RConn1 -- Source_For_LF/RConn1 -- Load Flow Bus/LConn1

== system VSC_GFo_Fixed_Frequency_wi_LCL_v2017b/VSC00/Low Pass Filter ==
  Filter capacitance : powerlib/Elements/Three-Phase Series RLC Branch  LConnTagsString=A|B|C  RConnTagsString=A|B|C  BranchType=C  Resistance=0  Inductance=C_line(1)  Capacitance=Cf_pu*Cb  Measurements=Branch voltages
      settings: SourceProductName=Simscape Electrical
  Filter inductance : powerlib/Elements/Three-Phase Series RLC Branch  LConnTagsString=A|B|C  RConnTagsString=A|B|C  BranchType=L  Resistance=0  Inductance=Lf_pu*Lb  Capacitance=1e-6  Measurements=None
      settings: SourceProductName=Simscape Electrical
  Ground : powerlib/Elements/Ground  LConnTagsString=a
      settings: SourceProductName=Simscape Electrical
  A : PMIOPort  Port=1  Side=Left
  a : PMIOPort  Port=2  Side=Right
  B : PMIOPort  Port=3  Side=Left
  b : PMIOPort  Port=4  Side=Right
  C : PMIOPort  Port=5  Side=Left
  c : PMIOPort  Port=6  Side=Right
  connections:
  Filter inductance/LConn3 -- C/RConn1
  c/RConn1 -- Filter inductance/RConn3 -- Filter capacitance/LConn3
  Ground/LConn1 -- Filter capacitance/RConn1 -- Filter capacitance/RConn2 -- Filter capacitance/RConn3
  Filter inductance/LConn2 -- B/RConn1
  Filter inductance/LConn1 -- A/RConn1
  Filter capacitance/LConn1 -- Filter inductance/RConn1 -- a/RConn1
  Filter capacitance/LConn2 -- Filter inductance/RConn2 -- b/RConn1

== system VSC_GFo_Fixed_Frequency_wi_LCL_v2017b/VSC00/Mean_model ==
  Uref : Inport
  Mean_model : Subsystem  Commented=on
  NOT1 : Logic  Operator=NOT  IconShape=distinctive  AllPortsSameDT=off  OutDataTypeStr=boolean
  Scope : Scope
  Step1 : Step  Time=Time_Step  SampleTime=Time_Step
  Three-Phase Breaker1 : powerlib/Elements/Three-Phase Breaker  InitialState=closed  SwitchA=on  SwitchB=on  SwitchC=on  SwitchTimes="[4/60  10/60]"  External=on  BreakerResistance=0.0001  SnubberResistance=1e6  SnubberCapacitance=inf  Measurements=None
      settings: SourceProductName=Simscape Electrical
  Three-Phase Breaker2 : powerlib/Elements/Three-Phase Breaker  InitialState=open  SwitchA=on  SwitchB=on  SwitchC=on  SwitchTimes="[4/60  10/60]"  External=on  BreakerResistance=0.0001  SnubberResistance=1e6  SnubberCapacitance=inf  Measurements=None
      settings: SourceProductName=Simscape Electrical
  Three-Phase Source : powerlib/Electrical Sources/Three-Phase Source  InternalConnection=Yg  VoltagePhases=off  Voltage=Vvsc0*Un1  PhaseAngle=Theta_vsc0  Voltage_phases=[25e3 25e3 25e3]/sqrt(3)  PhaseAngles_phases=[0 -120 +120]  Frequency=50  NonIdealSource=off  SpecifyImpedance=off  Resistance=0  Inductance=0  ShortCircuitLevel=100e6  BaseVoltage=VSC01_Un1  XRratio=7  BusType=swing  Pref=0.3  Qref=0  Prefabc=[10e3, 10e3, 10e3]  Qrefabc=[0, 0, 0]  Qmin=-Inf  Qmax=Inf
      settings: SourceProductName=Simscape Electrical
  Universal Bridge : powerlib/Power Electronics/Universal Bridge  Arms=3  SnubberResistance=1e5  SnubberCapacitance=inf  Device=Average-model based VSC  Ron=1e-3  Lon=0  ForwardVoltages="[  0  0  ]"  ForwardVoltage=0  GTOparameters=[ 10e-6 , 20e-6 ]  IGBTparameters=[ 1e-6 , 2e-6 ]  Measurements=None  Measurements_2=None  converterType=Rectifier
  Vdc : powerlib/Measurements/Voltage Measurement  PhasorSimulation=off  OutputType=Complex  PSBequivalent=0
      settings: SourceProductName=Simscape Electrical
  mp3 : Gain  Gain=2/VSC01_Udcb
  PhA : PMIOPort  Port=1  Side=Right
  PhB : PMIOPort  Port=2  Side=Right
  PhC : PMIOPort  Port=3  Side=Right
  Vdc+ : PMIOPort  Port=4  Side=Left
  Vdc- : PMIOPort  Port=5  Side=Left
  wires:
  Vdc/1 -> Scope/1
  Uref/1 -> mp3/1
  mp3/1 -> Universal Bridge/1
  Step1/1 -> Three-Phase Breaker2/1, NOT1/1
  NOT1/1 -> Three-Phase Breaker1/1
  connections:
  Vdc-/RConn1 -- Universal Bridge/RConn2 -- Vdc/LConn2
  Vdc+/RConn1 -- Universal Bridge/RConn1 -- Vdc/LConn1
  Three-Phase Source/RConn3 -- Three-Phase Breaker1/RConn3
  Three-Phase Source/RConn2 -- Three-Phase Breaker1/RConn2
  Three-Phase Source/RConn1 -- Three-Phase Breaker1/RConn1
  Universal Bridge/LConn3 -- Three-Phase Breaker2/RConn3
  Universal Bridge/LConn2 -- Three-Phase Breaker2/RConn2
  Universal Bridge/LConn1 -- Three-Phase Breaker2/RConn1
  PhC/RConn1 -- Three-Phase Breaker1/LConn3 -- Three-Phase Breaker2/LConn3
  PhB/RConn1 -- Three-Phase Breaker1/LConn2 -- Three-Phase Breaker2/LConn2
  PhA/RConn1 -- Three-Phase Breaker1/LConn1 -- Three-Phase Breaker2/LConn1

== system VSC_GFo_Fixed_Frequency_wi_LCL_v2017b/VSC00/PLL ==
  v_pcc : Inport
  0 - Vd1 : Gain  Gain=1/Vb  SaturateOnIntegerOverflow=on  OutDataTypeStr=Inherit: Same as input  ParamDataTypeStr=Inherit: Same as input
  Correcteur PI : Subsystem
  Scope : Scope
  Terminator : Terminator
  abc --> dq : Subsystem
  delta_PLL : Outport
  w_PLL : Outport  Port=2
  wires:
  v_pcc/1 -> 0 - Vd1/1
  0 - Vd1/1 -> abc --> dq/1(vpcc_abc)
  abc --> dq/2(vpcc_q) -> Scope/1, Correcteur PI/1(In1)
  Correcteur PI/1(w_PLL) -> w_PLL/1
  abc --> dq/1(vpcc_d) -> Terminator/1
  Correcteur PI/2(delta_theta) -> delta_PLL/1, abc --> dq/2(Theta)

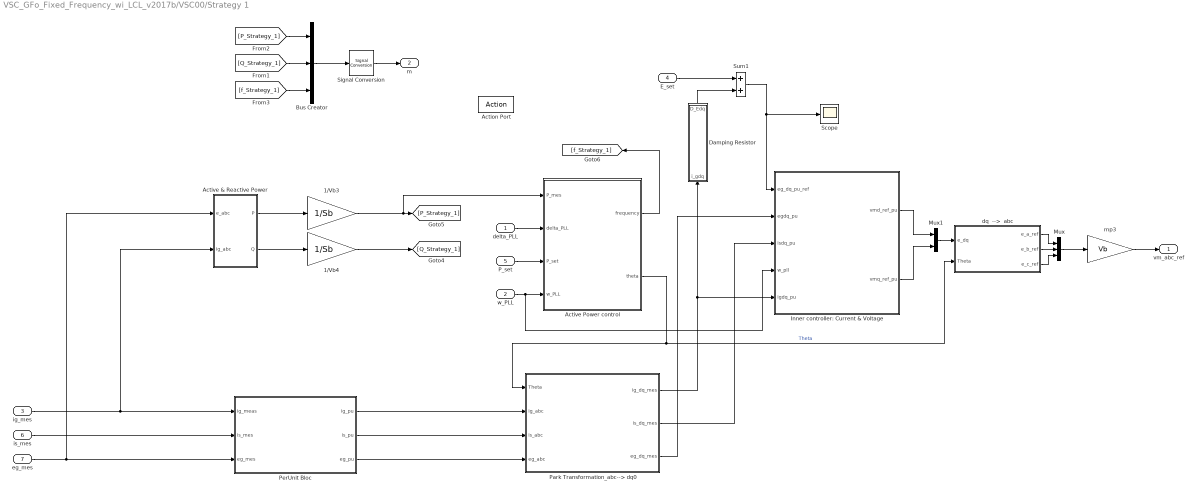
== system VSC_GFo_Fixed_Frequency_wi_LCL_v2017b/VSC00/Strategy 1 ==
  delta_PLL : Inport
  w_PLL : Inport  Port=2
  ig_mes : Inport  Port=3
  E_set : Inport  Port=4
  P_set : Inport  Port=5
  is_mes : Inport  Port=6
  eg_mes : Inport  Port=7
  Action Port : ActionPort  ActionType=case
  " Active & Reactive Power" : Subsystem  DialogController=POWERSYS.PowerSysDialog
  1/Vb3 : Gain  Gain=1/Sb
  1/Vb4 : Gain  Gain=1/Sb
  Active Power control : Subsystem
  Bus Creator : BusCreator  Inputs=3
  Damping Resistor : Subsystem
  "Inner controller: Current & Voltage " : Subsystem
  Mux : Mux  Inputs=3
  Mux1 : Mux  Inputs=2
  Park Transformation_abc--> dq0 : Subsystem
  PerUnit Bloc : Subsystem
  Scope : Scope
  Signal Conversion : SignalConversion  OverrideOpt=off
  Sum1 : Sum
  "dq  -->  abc " : Subsystem
  mp3 : Gain  Gain=Vb
  vm_abc_ref : Outport
  m : Outport  Port=2
  wires:
  Bus Creator/1 -> Signal Conversion/1
  Signal Conversion/1 -> m/1
  [P_Strategy_1] -> Bus Creator/1
  [Q_Strategy_1] -> Bus Creator/2
  [f_Strategy_1] -> Bus Creator/3
  mp3/1 -> vm_abc_ref/1
  "dq  -->  abc "/3(e_c_ref) -> Mux/3
  " Active & Reactive Power"/1(P) -> 1/Vb3/1
  " Active & Reactive Power"/2(Q) -> 1/Vb4/1
  1/Vb3/1 -> Active Power control/1(P_mes), [P_Strategy_1]
  Mux/1 -> mp3/1
  1/Vb4/1 -> [Q_Strategy_1]
  "dq  -->  abc "/2(e_b_ref) -> Mux/2
  "dq  -->  abc "/1(e_a_ref) -> Mux/1
  delta_PLL/1 -> Active Power control/2(delta_PLL)
  P_set/1 -> Active Power control/3(P_set)
  Mux1/1 -> "dq  -->  abc "/1(e_dq)
  "Inner controller: Current & Voltage "/1(vmd_ref_pu) -> Mux1/1
  "Inner controller: Current & Voltage "/2(vmq_ref_pu) -> Mux1/2
  E_set/1 -> Sum1/1
  Sum1/1 -> Scope/1, "Inner controller: Current & Voltage "/1(eg_dq_pu_ref)
  Active Power control/2(theta) -> "dq  -->  abc "/2(Theta), Park Transformation_abc--> dq0/1(Theta)  "Theta"
  Active Power control/1(frequency) -> [f_Strategy_1]
  Park Transformation_abc--> dq0/1(ig_dq_mes) -> Damping Resistor/1(i_gdq), "Inner controller: Current & Voltage "/5(igdq_pu)
  Park Transformation_abc--> dq0/3(eg_dq_mes) -> "Inner controller: Current & Voltage "/2(egdq_pu)
  Park Transformation_abc--> dq0/2(is_dq_mes) -> "Inner controller: Current & Voltage "/3("isdq_pu ")
  w_PLL/1 -> "Inner controller: Current & Voltage "/4(w_pll), Active Power control/4(w_PLL)
  is_mes/1 -> PerUnit Bloc/2(is_mes)
  eg_mes/1 -> " Active & Reactive Power"/1(e_abc), PerUnit Bloc/3(eg_mes)
  PerUnit Bloc/1(ig_pu) -> Park Transformation_abc--> dq0/2(ig_abc)
  PerUnit Bloc/2(is_pu) -> Park Transformation_abc--> dq0/3(is_abc)
  PerUnit Bloc/3(eg_pu) -> Park Transformation_abc--> dq0/4(eg_abc)
  Damping Resistor/1("D_Edq ") -> Sum1/2
  ig_mes/1 -> " Active & Reactive Power"/2(Ig_abc), PerUnit Bloc/1(ig_meas)

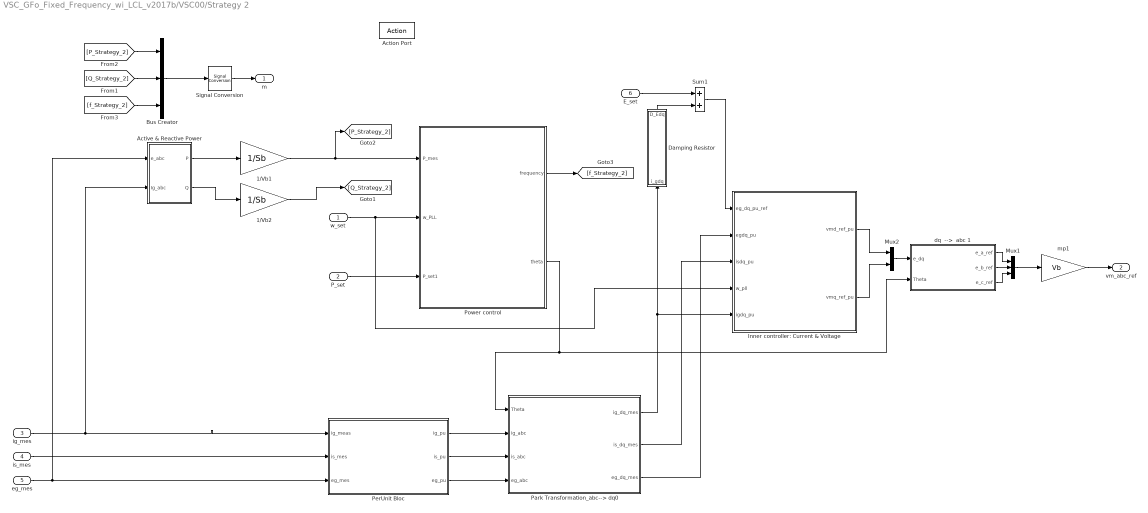
== system VSC_GFo_Fixed_Frequency_wi_LCL_v2017b/VSC00/Strategy 2 ==
  w_set : Inport
  P_set : Inport  Port=2
  ig_mes : Inport  Port=3
  is_mes : Inport  Port=4
  eg_mes : Inport  Port=5
  E_set : Inport  Port=6
  Action Port : ActionPort  ActionType=case
  " Active & Reactive Power" : Subsystem  DialogController=POWERSYS.PowerSysDialog
  1/Vb1 : Gain  Gain=1/Sb
  1/Vb2 : Gain  Gain=1/Sb
  Bus Creator : BusCreator  Inputs=3
  Damping Resistor : Subsystem
  "Inner controller: Current & Voltage " : Subsystem
  Mux1 : Mux  Inputs=3
  Mux2 : Mux  Inputs=2
  Park Transformation_abc--> dq0 : Subsystem
  PerUnit Bloc : Subsystem
  Power control : Subsystem
  Signal Conversion : SignalConversion  OverrideOpt=off
  Sum1 : Sum
  dq  -->  abc 1 : Subsystem
  mp1 : Gain  Gain=Vb
  m : Outport
  vm_abc_ref : Outport  Port=2
  wires:
  w_set/1 -> "Inner controller: Current & Voltage "/4(w_pll), Power control/2(w_PLL)
  P_set/1 -> Power control/3(P_set1)
  1/Vb1/1 -> [P_Strategy_2], Power control/1(P_mes)
  1/Vb2/1 -> [Q_Strategy_2]
  [Q_Strategy_2] -> Bus Creator/2
  Bus Creator/1 -> Signal Conversion/1
  [P_Strategy_2] -> Bus Creator/1
  [f_Strategy_2] -> Bus Creator/3
  Signal Conversion/1 -> m/1
  Power control/1(frequency) -> [f_Strategy_2]
  " Active & Reactive Power"/2(Q) -> 1/Vb2/1
  " Active & Reactive Power"/1(P) -> 1/Vb1/1
  PerUnit Bloc/2(is_pu) -> Park Transformation_abc--> dq0/3(is_abc)
  is_mes/1 -> PerUnit Bloc/2(is_mes)
  PerUnit Bloc/3(eg_pu) -> Park Transformation_abc--> dq0/4(eg_abc)
  ig_mes/1 -> " Active & Reactive Power"/2(Ig_abc), PerUnit Bloc/1(ig_meas)
  eg_mes/1 -> " Active & Reactive Power"/1(e_abc), PerUnit Bloc/3(eg_mes)
  PerUnit Bloc/1(ig_pu) -> Park Transformation_abc--> dq0/2(ig_abc)
  dq  -->  abc 1/3(e_c_ref) -> Mux1/3
  "Inner controller: Current & Voltage "/1(vmd_ref_pu) -> Mux2/1
  dq  -->  abc 1/2(e_b_ref) -> Mux1/2
  Mux1/1 -> mp1/1
  Sum1/1 -> "Inner controller: Current & Voltage "/1(eg_dq_pu_ref)
  dq  -->  abc 1/1(e_a_ref) -> Mux1/1
  mp1/1 -> vm_abc_ref/1
  E_set/1 -> Sum1/1
  "Inner controller: Current & Voltage "/2(vmq_ref_pu) -> Mux2/2
  Mux2/1 -> dq  -->  abc 1/1(e_dq)
  Damping Resistor/1("D_Edq ") -> Sum1/2
  Park Transformation_abc--> dq0/1(ig_dq_mes) -> "Inner controller: Current & Voltage "/5(igdq_pu), Damping Resistor/1(i_gdq)
  Park Transformation_abc--> dq0/2(is_dq_mes) -> "Inner controller: Current & Voltage "/3("isdq_pu ")
  Park Transformation_abc--> dq0/3(eg_dq_mes) -> "Inner controller: Current & Voltage "/2(egdq_pu)
  Power control/2(theta) -> dq  -->  abc 1/2(Theta), Park Transformation_abc--> dq0/1(Theta)

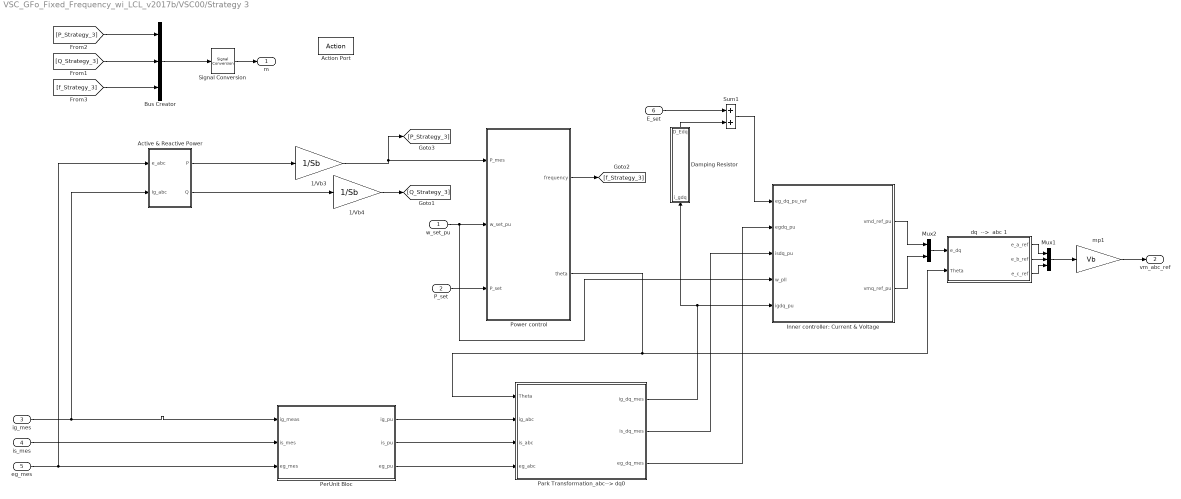
== system VSC_GFo_Fixed_Frequency_wi_LCL_v2017b/VSC00/Strategy 3 ==
  w_set_pu : Inport
  P_set : Inport  Port=2
  ig_mes : Inport  Port=3
  is_mes : Inport  Port=4
  eg_mes : Inport  Port=5
  E_set : Inport  Port=6
  Action Port : ActionPort  ActionType=case
  " Active & Reactive Power" : Subsystem  DialogController=POWERSYS.PowerSysDialog
  1/Vb3 : Gain  Gain=1/Sb
  1/Vb4 : Gain  Gain=1/Sb
  Bus Creator : BusCreator  Inputs=3
  Damping Resistor : Subsystem
  "Inner controller: Current & Voltage " : Subsystem
  Mux1 : Mux  Inputs=3
  Mux2 : Mux  Inputs=2
  Park Transformation_abc--> dq0 : Subsystem
  PerUnit Bloc : Subsystem
  Power control : Subsystem
  Signal Conversion : SignalConversion  OverrideOpt=off
  Sum1 : Sum
  dq  -->  abc 1 : Subsystem
  mp1 : Gain  Gain=Vb
  m : Outport
  vm_abc_ref : Outport  Port=2
  wires:
  Signal Conversion/1 -> m/1
  [Q_Strategy_3] -> Bus Creator/2
  Bus Creator/1 -> Signal Conversion/1
  [P_Strategy_3] -> Bus Creator/1
  [f_Strategy_3] -> Bus Creator/3
  1/Vb3/1 -> [P_Strategy_3], Power control/1(P_mes)
  " Active & Reactive Power"/2(Q) -> 1/Vb4/1
  w_set_pu/1 -> "Inner controller: Current & Voltage "/4(w_pll), Power control/2(w_set_pu)
  1/Vb4/1 -> [Q_Strategy_3]
  " Active & Reactive Power"/1(P) -> 1/Vb3/1
  eg_mes/1 -> " Active & Reactive Power"/1(e_abc), PerUnit Bloc/3(eg_mes)
  P_set/1 -> Power control/3(P_set)
  Power control/1(frequency) -> [f_Strategy_3]
  ig_mes/1 -> " Active & Reactive Power"/2(Ig_abc), PerUnit Bloc/1(ig_meas)
  PerUnit Bloc/3(eg_pu) -> Park Transformation_abc--> dq0/4(eg_abc)
  PerUnit Bloc/1(ig_pu) -> Park Transformation_abc--> dq0/2(ig_abc)
  is_mes/1 -> PerUnit Bloc/2(is_mes)
  PerUnit Bloc/2(is_pu) -> Park Transformation_abc--> dq0/3(is_abc)
  "Inner controller: Current & Voltage "/1(vmd_ref_pu) -> Mux2/1
  dq  -->  abc 1/3(e_c_ref) -> Mux1/3
  mp1/1 -> vm_abc_ref/1
  Mux1/1 -> mp1/1
  Damping Resistor/1("D_Edq ") -> Sum1/2
  dq  -->  abc 1/2(e_b_ref) -> Mux1/2
  dq  -->  abc 1/1(e_a_ref) -> Mux1/1
  Mux2/1 -> dq  -->  abc 1/1(e_dq)
  "Inner controller: Current & Voltage "/2(vmq_ref_pu) -> Mux2/2
  E_set/1 -> Sum1/1
  Sum1/1 -> "Inner controller: Current & Voltage "/1(eg_dq_pu_ref)
  Park Transformation_abc--> dq0/1(ig_dq_mes) -> "Inner controller: Current & Voltage "/5(igdq_pu), Damping Resistor/1(i_gdq)
  Power control/2(theta) -> Park Transformation_abc--> dq0/1(Theta), dq  -->  abc 1/2(Theta)
  Park Transformation_abc--> dq0/2(is_dq_mes) -> "Inner controller: Current & Voltage "/3("isdq_pu ")
  Park Transformation_abc--> dq0/3(eg_dq_mes) -> "Inner controller: Current & Voltage "/2(egdq_pu)

== system VSC_GFo_Fixed_Frequency_wi_LCL_v2017b/Voltage Source/Mean_model ==
  u_abc : Inport
  Controlled Voltage Source1 : powerlib/Electrical Sources/Controlled Voltage Source  Initialize=on  Source_Type=AC  Amplitude=e0*sqrt(2)  Phase=0  Frequency=fb  Measurements=None
      settings: SourceProductName=Simscape Electrical
  Controlled Voltage Source2 : powerlib/Electrical Sources/Controlled Voltage Source  Initialize=on  Source_Type=AC  Amplitude=e0*sqrt(2)  Phase=-240  Frequency=fb  Measurements=None
      settings: SourceProductName=Simscape Electrical
  Controlled Voltage Source4 : powerlib/Electrical Sources/Controlled Voltage Source  Initialize=on  Source_Type=AC  Amplitude=e0*sqrt(2)  Phase=-120  Frequency=fb  Measurements=None
      settings: SourceProductName=Simscape Electrical
  Demux : Demux  Outputs=3
  Ground2 : powerlib/Elements/Ground  LConnTagsString=a
      settings: SourceProductName=Simscape Electrical
  A : PMIOPort  Port=1  Side=Right
  B : PMIOPort  Port=2  Side=Right
  C : PMIOPort  Port=3  Side=Right
  wires:
  u_abc/1 -> Demux/1
  Demux/2 -> Controlled Voltage Source4/1
  Demux/3 -> Controlled Voltage Source2/1
  Demux/1 -> Controlled Voltage Source1/1
  connections:
  Controlled Voltage Source4/LConn1 -- Controlled Voltage Source1/LConn1 -- Controlled Voltage Source2/LConn1 -- Ground2/LConn1
  Controlled Voltage Source2/RConn1 -- C/RConn1
  Controlled Voltage Source4/RConn1 -- B/RConn1
  Controlled Voltage Source1/RConn1 -- A/RConn1

== system VSC_GFo_Fixed_Frequency_wi_LCL_v2017b/Voltage Source/Voltage generation ==
  E_set : Inport
  Mux : Mux  Inputs=3
  Voltage generation : Subsystem
  pu --> SI : Subsystem
  vg_abc : Outport
  wires:
  pu --> SI/1(e_a_SI) -> Mux/1
  Voltage generation/3(v_c) -> pu --> SI/3(e_c_pu)
  Mux/1 -> vg_abc/1
  pu --> SI/3(e_c_SI) -> Mux/3
  pu --> SI/2(e_b_SI) -> Mux/2
  Voltage generation/1(v_a) -> pu --> SI/1(e_a_pu)
  Voltage generation/2(v_b) -> pu --> SI/2(e_b_pu)
  E_set/1 -> Voltage generation/1(E_set)

== system VSC_GFo_Fixed_Frequency_wi_LCL_v2017b/VSC00/Mean_model/Mean_model ==
  In_A : Inport
  In_B : Inport  Port=2
  In_C : Inport  Port=3
  Controlled Voltage Source1 : powerlib/Electrical Sources/Controlled Voltage Source  Initialize=on  Source_Type=AC  Amplitude=Vvsc0*Vb  Phase=Theta_vsc0-120  Frequency=fb  Measurements=None
  Controlled Voltage Source2 : powerlib/Electrical Sources/Controlled Voltage Source  Initialize=on  Source_Type=AC  Amplitude=Vvsc0*Vb  Phase=Theta_vsc0+120  Frequency=fb  Measurements=None
  Controlled Voltage Source3 : powerlib/Electrical Sources/Controlled Voltage Source  Initialize=on  Source_Type=AC  Amplitude=Vvsc0*Vb  Phase=Theta_vsc0  Frequency=fb  Measurements=Voltage
  Ground : powerlib/Elements/Ground  LConnTagsString=a
  A : PMIOPort  Port=1  Side=Right
  B : PMIOPort  Port=2  Side=Right
  C : PMIOPort  Port=3  Side=Right
  wires:
  In_A/1 -> Controlled Voltage Source3/1
  In_C/1 -> Controlled Voltage Source2/1
  In_B/1 -> Controlled Voltage Source1/1
  connections:
  B/RConn1 -- Controlled Voltage Source1/RConn1
  Controlled Voltage Source2/LConn1 -- Ground/LConn1 -- Controlled Voltage Source3/LConn1 -- Controlled Voltage Source1/LConn1
  Controlled Voltage Source3/RConn1 -- A/RConn1
  C/RConn1 -- Controlled Voltage Source2/RConn1
